simulink model "AdaptiveFilt_Product"  (R2022b)
settings: Solver=VariableStepAuto  StartTime=0.0  StopTime=inf  MaxStep=1e-3  RelTol=1e-6
libraries: commchan3 x1
settings Model: Creator=Ceribro  LastModifiedBy=Ceribro

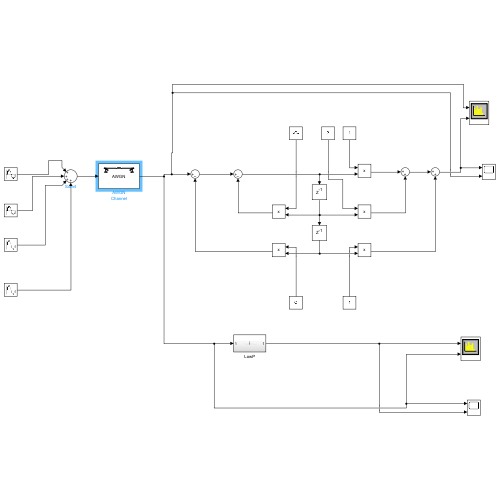
[thumbnail: Simulink's stored preview of the top-level diagram]
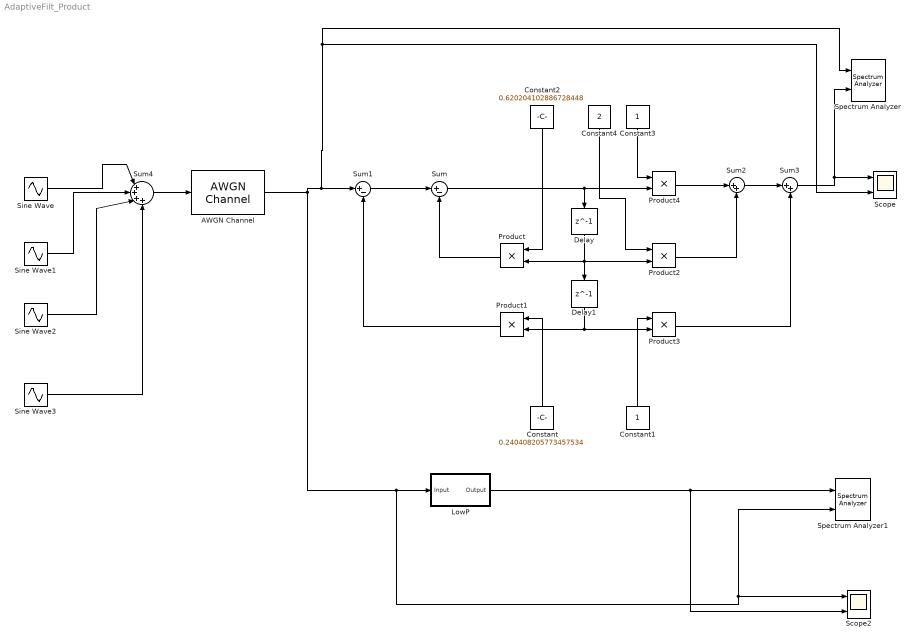
== system AdaptiveFilt_Product ==
  AWGN Channel : commchan3/AWGN Channel  InputProcessing=Columns as channels (frame based)  seed=67  noiseMode="Signal to noise ratio  (SNR)"  EbNodB=10  EsNodB=10  SNRdB=-22  bitsPerSym=1  Ps=1  Tsym=1  variance=1
  Constant : Constant  Value=0.240408205773457534
  Constant1 : Constant
  Constant2 : Constant  Value=0.620204102886728448
  Constant3 : Constant
  Constant4 : Constant  Value=2
  Delay : Delay  DelayLength=1  InitialCondition=0
  Delay1 : Delay  DelayLength=1  InitialCondition=0
  LowP : Subsystem  Tag=FilterWizardSubSystem
      settings: ErrorFcn=dspFilterRealizedInBasicElemsAlgLoopErrFcnCallback
  Product{,1..4} (5 alike) : Product
  Scope : Scope  NumInputPorts=2
  Scope2 : Scope  NumInputPorts=2
  Sine Wave : Sin  Frequency=1000*2*pi  SampleTime=1/44.1e3
  Sine Wave1 : Sin  Frequency=15000*2*pi  SampleTime=1/44.1e3
  Sine Wave2 : Sin  Frequency=18000*2*pi  SampleTime=1/44.1e3
  Sine Wave3 : Sin  Frequency=7000*2*pi  SampleTime=1/44.1e3
  Spectrum Analyzer : SpectrumAnalyzer  NumInputPorts=2
  Spectrum Analyzer1 : SpectrumAnalyzer  NumInputPorts=2
  Sum : Sum  Inputs=|+-
  Sum1 : Sum  Inputs=|+-
  Sum2 : Sum  Inputs=|++
  Sum3 : Sum  Inputs=|++
  Sum4 : Sum  Inputs=|++++
  wires:
  Product4/1 -> Sum2/1
  Sum2/1 -> Sum3/1
  Sum1/1 -> Sum/1
  Delay1/1 -> Product3/2, Product1/2
  Delay/1 -> Product2/2, Product/2, Delay1/1
  Sum/1 -> Product4/2, Delay/1
  Product2/1 -> Sum2/2
  Product3/1 -> Sum3/2
  Product1/1 -> Sum1/2
  Product/1 -> Sum/2
  Constant/1 -> Product1/1
  Constant1/1 -> Product3/1
  Constant3/1 -> Product4/1
  Constant2/1 -> Product/1
  Constant4/1 -> Product2/1
  Sum3/1 -> Spectrum Analyzer/2, Scope/1
  Sine Wave/1 -> Sum4/1
  Sine Wave1/1 -> Sum4/2
  Sum4/1 -> AWGN Channel/1
  Sine Wave2/1 -> Sum4/3
  LowP/1(Output) -> Scope2/2, Spectrum Analyzer1/1
  Sine Wave3/1 -> Sum4/4
  AWGN Channel/1 -> Scope/2, Spectrum Analyzer/1, Sum1/1, LowP/1(Input), Spectrum Analyzer1/2, Scope2/1

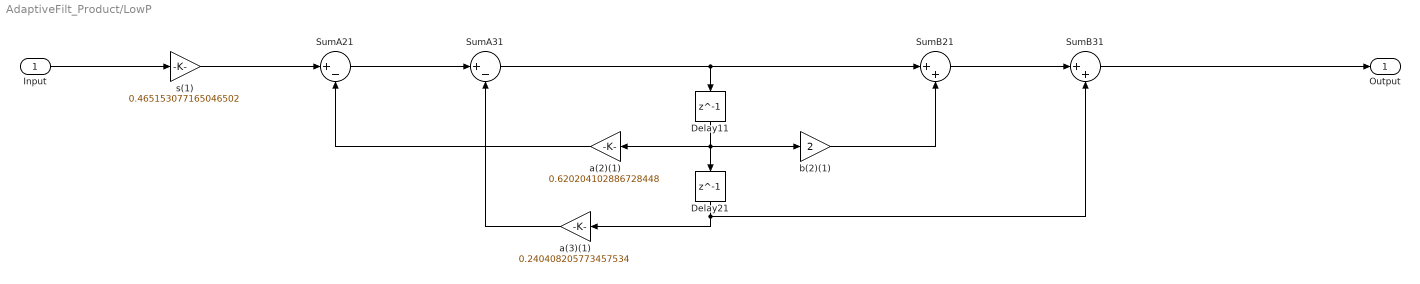
== system AdaptiveFilt_Product/LowP ==
  Input : Inport
  Delay11 : Delay  DelayLength=1  InitialCondition=0
  Delay21 : Delay  DelayLength=1  InitialCondition=0
  SumA21 : Sum  Inputs=|+-  RndMeth=Nearest  SaturateOnIntegerOverflow=on  OutDataTypeStr=Inherit: Same as first input
  SumA31 : Sum  Inputs=|+-  RndMeth=Nearest  SaturateOnIntegerOverflow=on  OutDataTypeStr=Inherit: Same as first input
  SumB21 : Sum  Inputs=|++  RndMeth=Nearest  SaturateOnIntegerOverflow=on  OutDataTypeStr=Inherit: Same as first input
  SumB31 : Sum  Inputs=|++  RndMeth=Nearest  SaturateOnIntegerOverflow=on  OutDataTypeStr=Inherit: Same as first input
  a(2)(1) : Gain  Gain=0.620204102886728448  ParamDataTypeStr=double  RndMeth=Nearest  SaturateOnIntegerOverflow=on  OutDataTypeStr=Inherit: Same as input
  a(3)(1) : Gain  Gain=0.240408205773457534  ParamDataTypeStr=double  RndMeth=Nearest  SaturateOnIntegerOverflow=on  OutDataTypeStr=Inherit: Same as input
  b(2)(1) : Gain  Gain=2  ParamDataTypeStr=double  RndMeth=Nearest  SaturateOnIntegerOverflow=on  OutDataTypeStr=Inherit: Same as input
  s(1) : Gain  Gain=0.465153077165046502  ParamDataTypeStr=double  RndMeth=Nearest  SaturateOnIntegerOverflow=on  OutDataTypeStr=Inherit: Same as input
  Output : Outport
  wires:
  Input/1 -> s(1)/1
  s(1)/1 -> SumA21/1
  SumA21/1 -> SumA31/1
  SumA31/1 -> SumB21/1, Delay11/1
  SumB21/1 -> SumB31/1
  SumB31/1 -> Output/1
  a(2)(1)/1 -> SumA21/2
  Delay11/1 -> a(2)(1)/1, b(2)(1)/1, Delay21/1
  b(2)(1)/1 -> SumB21/2
  a(3)(1)/1 -> SumA31/2
  Delay21/1 -> a(3)(1)/1, SumB31/2
